simulink library "SimscapeMacros"  (R2016a)
settings: Solver=ode45  StartTime=0.0  StopTime=10.0  RelTol=1e-3
libraries: fl_lib x9, nesl_utility x3
settings Model: Creator=Peter  LastModifiedBy=Peter
settings DataIOCC: LimitDataPoints=on
settings DebuggingCC: AllowSymbolicDim=off

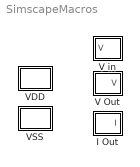
== system SimscapeMacros ==
  I Out : Subsystem
  V Out : Subsystem
  V in : Subsystem
  VDD : Subsystem
  VSS : Subsystem

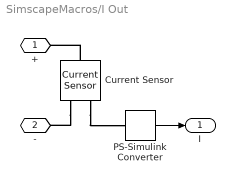
== system SimscapeMacros/I Out ==
  Current Sensor : fl_lib/Electrical/Electrical Sensors/Current Sensor
  PS-Simulink Converter : nesl_utility/PS-Simulink Converter  PhysicalDomain=network_engine_domain  SubClassName=ps_output  LeftPortType=input  RightPortType=output  PseudoPeriodic=off  Frequencies=[]  Unit=A  AffineConversion=off
  + : PMIOPort  Port=1  Side=Left
  - : PMIOPort  Port=2  Side=Left
  I : Outport
  wires:
  PS-Simulink Converter/1 -> I/1
  connections:
  Current Sensor/RConn2 -- -/RConn1
  Current Sensor/LConn1 -- +/RConn1
  Current Sensor/RConn1 -- PS-Simulink Converter/LConn1

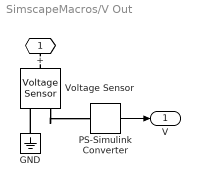
== system SimscapeMacros/V Out ==
  GND : fl_lib/Electrical/Electrical Elements/Electrical Reference
  PS-Simulink Converter : nesl_utility/PS-Simulink Converter  PhysicalDomain=network_engine_domain  SubClassName=ps_output  LeftPortType=input  RightPortType=output  PseudoPeriodic=off  Frequencies=[]  Unit=V  AffineConversion=off
  Voltage Sensor : fl_lib/Electrical/Electrical Sensors/Voltage Sensor
  + : PMIOPort  Port=1  Side=Left
  V : Outport
  wires:
  PS-Simulink Converter/1 -> V/1
  connections:
  Voltage Sensor/RConn1 -- PS-Simulink Converter/LConn1
  Voltage Sensor/LConn1 -- +/RConn1
  GND/LConn1 -- Voltage Sensor/RConn2

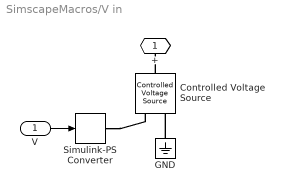
== system SimscapeMacros/V in ==
  V : Inport
  Controlled Voltage Source : fl_lib/Electrical/Electrical Sources/Controlled Voltage Source
  GND : fl_lib/Electrical/Electrical Elements/Electrical Reference
  Simulink-PS Converter : nesl_utility/Simulink-PS Converter  PhysicalDomain=network_engine_domain  SubClassName=ps_input  LeftPortType=input  RightPortType=output  PseudoPeriodic=off  Frequencies=[]  NoiseDistribution=none  NoiseParameters=[]  Unit=V  AffineConversion=off  InputFiltering=off  SimscapeFilterOrder=1  InputFilterTimeConstant=0.001  UdotUserProvided=1
  + : PMIOPort  Port=1  Side=Right
  wires:
  V/1 -> Simulink-PS Converter/1
  connections:
  Controlled Voltage Source/LConn1 -- +/RConn1
  Simulink-PS Converter/RConn1 -- Controlled Voltage Source/RConn1
  GND/LConn1 -- Controlled Voltage Source/RConn2

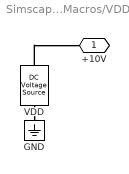
== system SimscapeMacros/VDD ==
  GND : fl_lib/Electrical/Electrical Elements/Electrical Reference
  VDD : fl_lib/Electrical/Electrical Sources/DC Voltage Source  v0=10 V
  +10V : PMIOPort  Port=1  Side=Right
  connections:
  VDD/LConn1 -- +10V/RConn1
  VDD/RConn1 -- GND/LConn1

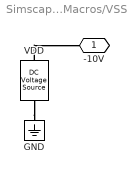
== system SimscapeMacros/VSS ==
  GND : fl_lib/Electrical/Electrical Elements/Electrical Reference
  VDD : fl_lib/Electrical/Electrical Sources/DC Voltage Source  v0=10 V
  -10V : PMIOPort  Port=1  Side=Right
  connections:
  VDD/LConn1 -- GND/LConn1
  VDD/RConn1 -- -10V/RConn1
